simulink model "FanSpd_VD"  (R2016b)
settings: configuration reference "CodeGenConfigSet" (kept outside this file)
values from neighbouring files (symbols this model uses):
  Fan_bswitchMonOn_C = Calibration.Parameter    [init_FanSpd_VD.m]
  Fan_facPT1_C = Calibration.Parameter    [init_FanSpd_VD.m]
  Fan_nEngMinPlaus_C = Calibration.Parameter    [init_FanSpd_VD.m]
  Fan_nevaluatedFlt_C = Calibration.Parameter    [init_FanSpd_VD.m]
  Fan_nMax_CUR = Calibration.Parameter    [init_FanSpd_VD.m]
  Fan_nMax_CURX = Calibration.Parameter    [init_FanSpd_VD.m]
  Fan_nMin_CUR = Calibration.Parameter    [init_FanSpd_VD.m]
  Fan_nMin_CURX = Calibration.Parameter    [init_FanSpd_VD.m]
  FanSpd_PWMINtimeroverflow_C = Calibration.Parameter    [init_FanSpd_VD.m]
  FanSpd_tiHighDebHiLo_C = Calibration.Parameter    [init_FanSpd_VD.m]
  FanSpd_tiHighDebLoHi_C = Calibration.Parameter    [init_FanSpd_VD.m]
  FanSpd_tiLonDebHiLo_C = Calibration.Parameter    [init_FanSpd_VD.m]
  FanSpd_tiLonDebLoHi_C = Calibration.Parameter    [init_FanSpd_VD.m]
  FanSpd_tiLowDebHiLo_C = Calibration.Parameter    [init_FanSpd_VD.m]
  FanSpd_tiLowDebLoHi_C = Calibration.Parameter    [init_FanSpd_VD.m]
undefined symbols (not defined in the file or in its folder): CEngDsT_tTransf_CURX, FanSpd_VD_DT
libraries: CXLib x4
settings Model: Creator=xinchangran  LastModifiedBy=xinchangran
settings ConfigSetRef: SourceLocation=Base Workspace

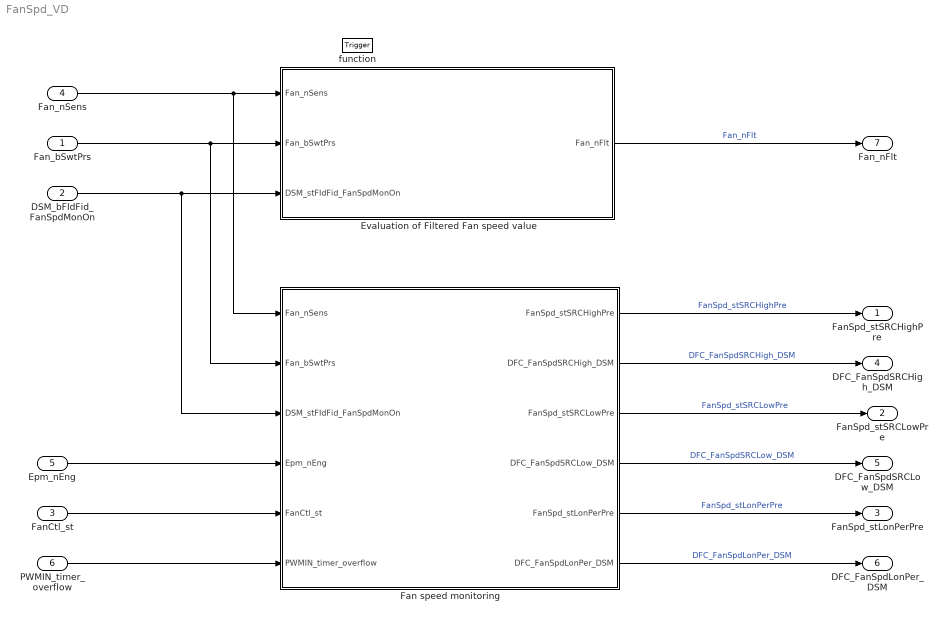
== system FanSpd_VD ==
  Fan_bSwtPrs : Inport  Description=Fan_bSwtPrs ==0 fan sensor is not installed/==1 sensor stalled  OutMin=0  OutMax=1  OutDataTypeStr=boolean
  DSM_bFIdFid_FanSpdMonOn : Inport  Description=monitoring signal  Port=2  OutMin=0  OutMax=255  OutDataTypeStr=State_uint8
  FanCtl_st : Inport  Port=3  OutMin=0  OutMax=255  OutDataTypeStr=State_uint8
  Fan_nSens : Inport  Tag=rpm  Description=Sensed fan speed  Port=4  OutMin=0  OutMax=32767  OutDataTypeStr=FanSpd_rpm
  Epm_nEng : Inport  Tag=rpm  Description=Engine speed  Port=5  OutMin=0  OutMax=6000  OutDataTypeStr=EngSpeed_rpm
  PWMIN_timer_overflow : Inport  Port=6  OutMin=0  OutMax=65535  OutDataTypeStr=State_uint16
  function : TriggerPort  TriggerType=function-call  VariantControl=Variant
  Evaluation of Filtered Fan speed value : Subsystem
  Fan speed monitoring : Subsystem
  FanSpd_stSRCHighPre : Outport  OutMin=0  OutMax=1  OutDataTypeStr=boolean
  FanSpd_stSRCLowPre : Outport  Port=2  OutMin=0  OutMax=1  OutDataTypeStr=boolean
  FanSpd_stLonPerPre : Outport  Port=3  OutMin=0  OutMax=1  OutDataTypeStr=boolean
  DFC_FanSpdSRCHigh_DSM : Outport  Description=after debouncing FanSpd_stSRCHighPre  Port=4  OutMin=0  OutMax=1  OutDataTypeStr=boolean
  DFC_FanSpdSRCLow_DSM : Outport  Description=after debouncing FanSpd_stSRCLowPre  Port=5  OutMin=0  OutMax=1  OutDataTypeStr=boolean
  DFC_FanSpdLonPer_DSM : Outport  Description=after debouncing FanSpd_stLonPerPre  Port=6  OutMin=0  OutMax=1  OutDataTypeStr=boolean
  Fan_nFlt : Outport  Tag=rpm  Port=7  OutMin=0  OutMax=32767  OutDataTypeStr=FanSpd_rpm
  wires:
  Fan_bSwtPrs/1 -> Evaluation of Filtered Fan speed value/2(Fan_bSwtPrs), Fan speed monitoring/2(Fan_bSwtPrs)
  DSM_bFIdFid_FanSpdMonOn/1 -> Evaluation of Filtered Fan speed value/3(DSM_stFIdFid_FanSpdMonOn), Fan speed monitoring/3(DSM_stFIdFid_FanSpdMonOn)
  Evaluation of Filtered Fan speed value/1(Fan_nFlt) -> Fan_nFlt/1  "Fan_nFlt"
  Epm_nEng/1 -> Fan speed monitoring/4(Epm_nEng)
  FanCtl_st/1 -> Fan speed monitoring/5(FanCtl_st)
  PWMIN_timer_overflow/1 -> Fan speed monitoring/6(PWMIN_timer_overflow)
  Fan speed monitoring/1(FanSpd_stSRCHighPre) -> FanSpd_stSRCHighPre/1  "FanSpd_stSRCHighPre"
  Fan speed monitoring/2(DFC_FanSpdSRCHigh_DSM) -> DFC_FanSpdSRCHigh_DSM/1  "DFC_FanSpdSRCHigh_DSM"
  Fan speed monitoring/4(DFC_FanSpdSRCLow_DSM) -> DFC_FanSpdSRCLow_DSM/1  "DFC_FanSpdSRCLow_DSM"
  Fan speed monitoring/5(FanSpd_stLonPerPre) -> FanSpd_stLonPerPre/1  "FanSpd_stLonPerPre"
  Fan speed monitoring/6(DFC_FanSpdLonPer_DSM) -> DFC_FanSpdLonPer_DSM/1  "DFC_FanSpdLonPer_DSM"
  Fan_nSens/1 -> Evaluation of Filtered Fan speed value/1(Fan_nSens), Fan speed monitoring/1(Fan_nSens)
  Fan speed monitoring/3(FanSpd_stSRCLowPre) -> FanSpd_stSRCLowPre/1  "FanSpd_stSRCLowPre"

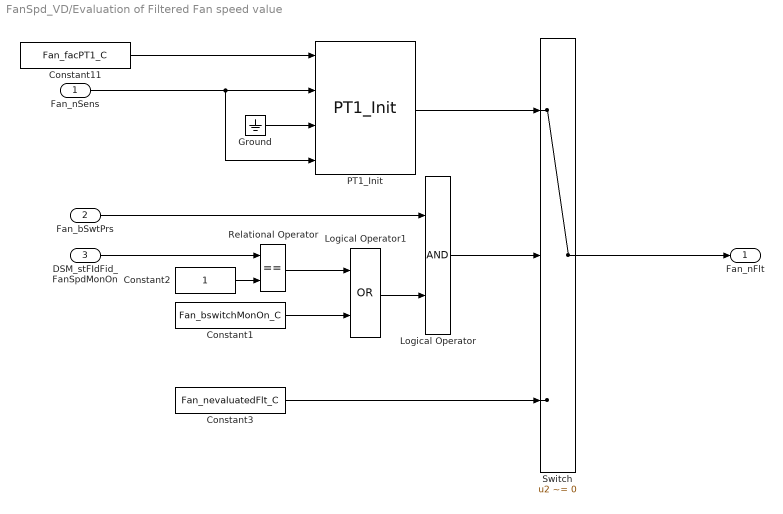
== system FanSpd_VD/Evaluation of Filtered Fan speed value ==
  Fan_nSens : Inport
  Fan_bSwtPrs : Inport  Port=2
  DSM_stFIdFid_FanSpdMonOn : Inport  Port=3
  Constant1 : Constant  Value=Fan_bswitchMonOn_C  SampleTime=-1
  Constant11 : Constant  Value=Fan_facPT1_C  SampleTime=-1
  Constant2 : Constant  OutDataTypeStr=Inherit: Inherit via back propagation
  Constant3 : Constant  Value=Fan_nevaluatedFlt_C  SampleTime=-1
  Ground : Ground
  Logical Operator : Logic  AllPortsSameDT=off  OutDataTypeStr=boolean
  Logical Operator1 : Logic  Operator=OR  AllPortsSameDT=off  OutDataTypeStr=boolean
  PT1_Init : CXLib/PT1_Init
  Relational Operator : RelationalOperator  Operator===  OutDataTypeStr=boolean  RndMeth=Simplest
  Switch : Switch  Criteria=u2 ~= 0  SaturateOnIntegerOverflow=on  InputSameDT=on
  Fan_nFlt : Outport
  wires:
  Constant11/1 -> PT1_Init/1
  Ground/1 -> PT1_Init/3
  Fan_nSens/1 -> PT1_Init/4, PT1_Init/2
  Fan_bSwtPrs/1 -> Logical Operator/1
  Constant3/1 -> Switch/3
  Switch/1 -> Fan_nFlt/1
  DSM_stFIdFid_FanSpdMonOn/1 -> Relational Operator/1
  Constant2/1 -> Relational Operator/2
  Relational Operator/1 -> Logical Operator1/1
  PT1_Init/1 -> Switch/1
  Constant1/1 -> Logical Operator1/2
  Logical Operator/1 -> Switch/2
  Logical Operator1/1 -> Logical Operator/2

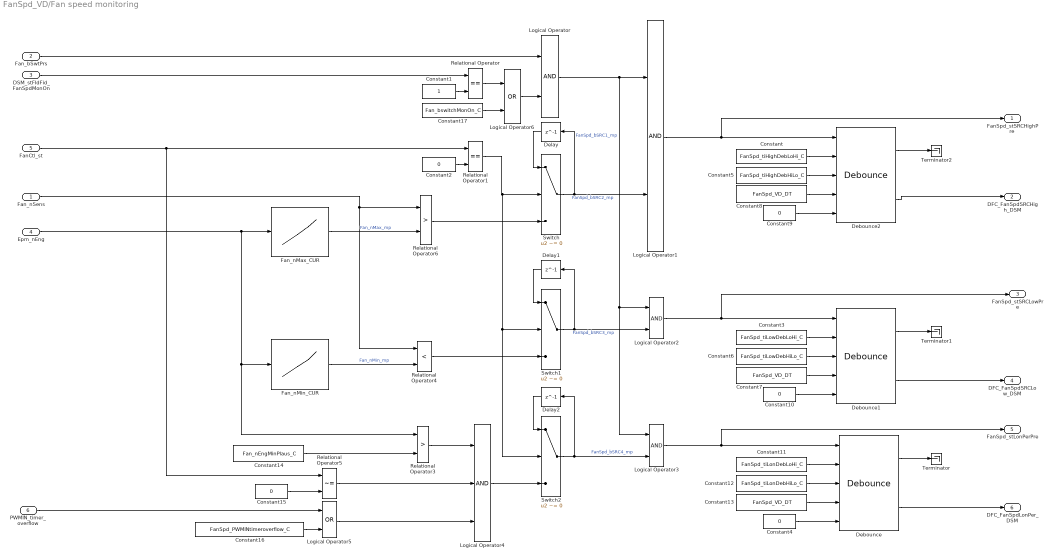
== system FanSpd_VD/Fan speed monitoring ==
  Fan_nSens : Inport
  Fan_bSwtPrs : Inport  Port=2
  DSM_stFIdFid_FanSpdMonOn : Inport  Port=3
  Epm_nEng : Inport  Port=4
  FanCtl_st : Inport  Port=5
  PWMIN_timer_overflow : Inport  Port=6
  Constant : Constant  Value=FanSpd_tiHighDebLoHi_C
  Constant1 : Constant  OutDataTypeStr=Inherit: Inherit via back propagation
  Constant{2,4,9..10,15} (5 alike) : Constant  Value=0  OutDataTypeStr=Inherit: Inherit via back propagation
  Constant11 : Constant  Value=FanSpd_tiLonDebLoHi_C
  Constant12 : Constant  Value=FanSpd_tiLonDebHiLo_C
  Constant13 : Constant  Value=FanSpd_VD_DT
  Constant14 : Constant  Value=Fan_nEngMinPlaus_C
  Constant16 : Constant  Value=FanSpd_PWMINtimeroverflow_C
  Constant17 : Constant  Value=Fan_bswitchMonOn_C  SampleTime=-1
  Constant3 : Constant  Value=FanSpd_tiLowDebLoHi_C
  Constant5 : Constant  Value=FanSpd_tiHighDebHiLo_C
  Constant6 : Constant  Value=FanSpd_tiLowDebHiLo_C
  Constant7 : Constant  Value=FanSpd_VD_DT
  Constant8 : Constant  Value=FanSpd_VD_DT
  Debounce : CXLib/Debounce
  Debounce1 : CXLib/Debounce
  Debounce2 : CXLib/Debounce
  Delay : Delay  DelayLength=1  InitialCondition=0
  Delay1 : Delay  DelayLength=1  InitialCondition=0
  Delay2 : Delay  DelayLength=1  InitialCondition=0
  Fan_nMax_CUR : Lookup_n-D  DialogController=Simulink.DDGSource  NumberOfTableDimensions=1  BreakpointsForDimension1=Fan_nMax_CURX  BreakpointsForDimension2=CEngDsT_tTransf_CURX  IndexSearchMethod=Linear search  BeginIndexSearchUsingPreviousIndexResult=on  Table=Fan_nMax_CUR  ExtrapMethod=Clip  UseLastTableValue=on  InternalRulePriority=Speed  OutDataTypeStr=Inherit: Inherit via back propagation  SaturateOnIntegerOverflow=on
  Fan_nMin_CUR : Lookup_n-D  DialogController=Simulink.DDGSource  NumberOfTableDimensions=1  BreakpointsForDimension1=Fan_nMin_CURX  BreakpointsForDimension2=CEngDsT_tTransf_CURX  IndexSearchMethod=Linear search  BeginIndexSearchUsingPreviousIndexResult=on  Table=Fan_nMin_CUR  ExtrapMethod=Clip  UseLastTableValue=on  InternalRulePriority=Speed  OutDataTypeStr=Inherit: Inherit via back propagation  SaturateOnIntegerOverflow=on
  Logical Operator{,1..3} (4 alike) : Logic  AllPortsSameDT=off  OutDataTypeStr=boolean
  Logical Operator4 : Logic  Inputs=3  AllPortsSameDT=off  OutDataTypeStr=boolean
  Logical Operator5 : Logic  Operator=OR  AllPortsSameDT=off  OutDataTypeStr=boolean
  Logical Operator6 : Logic  Operator=OR  AllPortsSameDT=off  OutDataTypeStr=boolean
  Relational Operator : RelationalOperator  Operator===  OutDataTypeStr=boolean  RndMeth=Simplest
  Relational Operator1 : RelationalOperator  Operator===  OutDataTypeStr=boolean  RndMeth=Simplest
  Relational Operator3 : RelationalOperator  Operator=>  OutDataTypeStr=boolean  RndMeth=Simplest
  Relational Operator4 : RelationalOperator  Operator=<  OutDataTypeStr=boolean  RndMeth=Simplest
  Relational Operator5 : RelationalOperator  Operator=~=  OutDataTypeStr=boolean  RndMeth=Simplest
  Relational Operator6 : RelationalOperator  Operator=>  OutDataTypeStr=boolean  RndMeth=Simplest
  Switch : Switch  Criteria=u2 ~= 0  InputSameDT=on
  Switch1 : Switch  Criteria=u2 ~= 0  InputSameDT=on
  Switch2 : Switch  Criteria=u2 ~= 0  InputSameDT=on
  Terminator : Terminator
  Terminator1 : Terminator
  Terminator2 : Terminator
  FanSpd_stSRCHighPre : Outport
  DFC_FanSpdSRCHigh_DSM : Outport  Port=2
  FanSpd_stSRCLowPre : Outport  Port=3
  DFC_FanSpdSRCLow_DSM : Outport  Port=4
  FanSpd_stLonPerPre : Outport  Port=5
  DFC_FanSpdLonPer_DSM : Outport  Port=6
  wires:
  Logical Operator4/1 -> Switch2/3
  Fan_nMax_CUR/1 -> Relational Operator6/2  "Fan_nMax_mp"
  Constant1/1 -> Relational Operator/2
  Debounce/1 -> Terminator/1
  Debounce1/1 -> Terminator1/1
  DSM_stFIdFid_FanSpdMonOn/1 -> Relational Operator/1
  Fan_bSwtPrs/1 -> Logical Operator/1
  Fan_nSens/1 -> Relational Operator4/1, Relational Operator6/1
  Constant2/1 -> Relational Operator1/2
  Constant5/1 -> Debounce2/3
  Constant/1 -> Debounce2/2
  Constant8/1 -> Debounce2/4
  Constant9/1 -> Debounce2/5
  Logical Operator1/1 -> Debounce2/1, FanSpd_stSRCHighPre/1
  Debounce2/2 -> DFC_FanSpdSRCHigh_DSM/1
  Constant6/1 -> Debounce1/3
  Constant10/1 -> Debounce1/5
  Constant3/1 -> Debounce1/2
  Fan_nMin_CUR/1 -> Relational Operator4/2  "Fan_nMin_mp"
  Delay1/1 -> Switch1/1
  Constant7/1 -> Debounce1/4
  Logical Operator2/1 -> Debounce1/1, FanSpd_stSRCLowPre/1
  Relational Operator4/1 -> Switch1/3
  Relational Operator1/1 -> Switch2/2, Switch1/2, Switch/2
  Switch1/1 -> Logical Operator2/2, Delay1/1  "FanSpd_bSRC3_mp"
  Debounce1/2 -> DFC_FanSpdSRCLow_DSM/1
  PWMIN_timer_overflow/1 -> Logical Operator5/1
  Relational Operator5/1 -> Logical Operator4/2
  FanCtl_st/1 -> Relational Operator5/1, Relational Operator1/1
  Constant15/1 -> Relational Operator5/2
  Delay/1 -> Switch/1
  Logical Operator/1 -> Logical Operator1/1, Logical Operator3/1, Logical Operator2/1  "FanSpd_bSRC1_mp"
  Logical Operator5/1 -> Logical Operator4/3
  Relational Operator6/1 -> Switch/3
  Relational Operator3/1 -> Logical Operator4/1
  Switch2/1 -> Delay2/1, Logical Operator3/2  "FanSpd_bSRC4_mp"
  Delay2/1 -> Switch2/1
  Debounce/2 -> DFC_FanSpdLonPer_DSM/1
  Logical Operator3/1 -> Debounce/1, FanSpd_stLonPerPre/1
  Epm_nEng/1 -> Relational Operator3/1, Fan_nMin_CUR/1, Fan_nMax_CUR/1
  Constant11/1 -> Debounce/2
  Constant4/1 -> Debounce/5
  Constant13/1 -> Debounce/4
  Constant14/1 -> Relational Operator3/2
  Constant12/1 -> Debounce/3
  Constant16/1 -> Logical Operator5/2
  Switch/1 -> Delay/1, Logical Operator1/2  "FanSpd_bSRC2_mp"
  Debounce2/1 -> Terminator2/1
  Constant17/1 -> Logical Operator6/2
  Relational Operator/1 -> Logical Operator6/1
  Logical Operator6/1 -> Logical Operator/2
